simulink model "openLoop"  (R2024a)
settings: Solver=VariableStepAuto  StartTime=0.0  StopTime=30  RelTol=1e-3
undefined symbols (not defined in the file or in its folder): initial_1, is501nmtbXaxis_simu
libraries: simulink x1
settings Model: Creator=b_ant  LastModifiedBy=b_ant

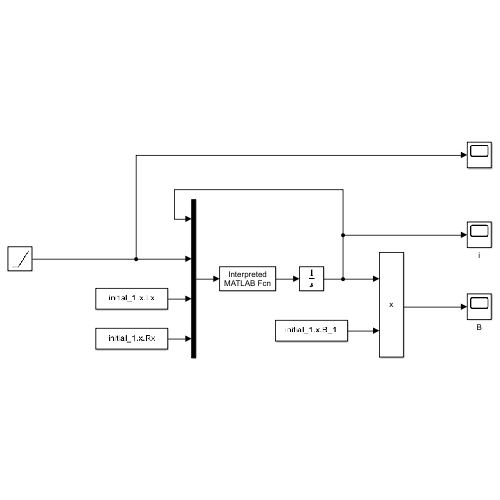
[thumbnail: Simulink's stored preview of the top-level diagram]
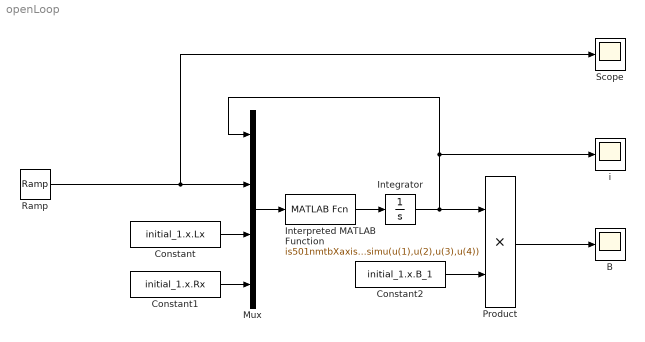
== system openLoop ==
  B : Scope
  Constant : Constant  Value=initial_1.x.Lx
  Constant1 : Constant  Value=initial_1.x.Rx
  Constant2 : Constant  Value=initial_1.x.B_1
  Integrator : Integrator
  Interpreted MATLAB Function : MATLABFcn  MATLABFcn=is501nmtbXaxis_simu(u(1),u(2),u(3),u(4))
  Mux : Mux
  Product : Product
  Ramp : simulink/Sources/Ramp  slope=-1  start=0  InitialOutput=15
  Scope : Scope
  i : Scope
  wires:
  Mux/1 -> Interpreted MATLAB Function/1
  Interpreted MATLAB Function/1 -> Integrator/1
  Integrator/1 -> Product/1, Mux/1, i/1
  Ramp/1 -> Scope/1, Mux/2
  Constant/1 -> Mux/3
  Constant1/1 -> Mux/4
  Constant2/1 -> Product/2
  Product/1 -> B/1
